simulink model "scdcstrctrlpidblock"  (Simulink 7.6)
settings: Solver=ode23s  StartTime=0  StopTime=60  RelTol=1e-3
libraries: simulink x1
settings Model: Creator=The MathWorks Inc.  BufferReuse=off
settings DataIOCC: InitialState=[311.267; 8.5695]  SaveOutput=off  SignalLogging=off  SaveTime=off  SignalLoggingName=logsOut
settings OptimizationCC: BooleanDataType=off  InlineParams=on  InlineInvariantSignals=on  BufferReuse=off  InitFltsAndDblsToZero=on
settings DebuggingCC: SaveWithParameterizedLinksMsg=none  CheckExecutionContextPreStartOutputMsg=on  CheckExecutionContextRuntimeOutputMsg=on  SignalResolutionControl=TryResolveAllWithWarning  SolverPrmCheckMsg=none  MultiTaskDSMMsg=warning  MultiTaskCondExecSysMsg=none  StrictBusMsg=None
settings HardwareCC: TargetUnknown=on
settings RTWCC: IncludeERTFirstTime=on
settings GRTTargetCC: TargetFcnLib=ansi_tfl_tmw.mat

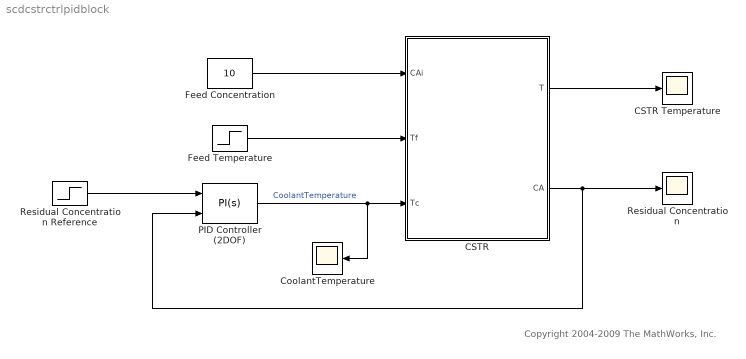
== system scdcstrctrlpidblock ==
  note: Copyright 2004-2009 The MathWorks, Inc.
  CSTR : Subsystem
  CSTR Temperature : Scope
      settings: YMin=300  YMax=750  SaveName=ScopeData2
  CoolantTemperature : Scope
      settings: YMin=300  YMax=750
  Feed Concentration : Constant  Value=10
  Feed Temperature : Step  Time=30  Before=300  After=305  SampleTime=0
  PID Controller (2DOF) : simulink/Continuous/PID Controller (2DOF)  DialogController=pidpack.PIDConfig.pidDDGCreate  DialogControllerArgs=DataTag0  SystemSampleTime=-1  Controller=PI  TimeDomain=Continuous-time  SampleTime=1  IntegratorMethod=Forward Euler  FilterMethod=Forward Euler  Form=Parallel  P=1  I=1  D=0  N=100  b=1  c=1  InitialConditionSource=internal  InitialConditionForIntegrator=300  InitialConditionForFilter=0  ExternalReset=none  ZeroCross=off  LimitOutput=off  UpperSaturationLimit=inf  LowerSaturationLimit=-inf  LinearizeAsGain=off  AntiWindupMode=none  Kb=1  TrackingMode=off  Kt=1  PParamMin=[ ]  PParamMax=[ ]  IParamMin=[ ]  IParamMax=[ ]  DParamMin=[ ]  DParamMax=[ ]  NParamMin=[ ]  NParamMax=[ ]  bParamMin=[ ]  bParamMax=[ ]  cParamMin=[ ]  cParamMax=[ ]  KbParamMin=[ ]  KbParamMax=[ ]  KtParamMin=[ ]  KtParamMax=[ ]  POutMin=[ ]  POutMax=[ ]  IOutMin=[ ]  IOutMax=[ ]  DOutMin=[ ]  DOutMax=[ ]  NOutMin=[ ]  NOutMax=[ ]  bOutMin=[ ]  bOutMax=[ ]  cOutMin=[ ]  cOutMax=[ ]  KbOutMin=[ ]  KbOutMax=[ ]  KtOutMin=[ ]  KtOutMax=[ ]  IntegratorOutMin=[ ]  IntegratorOutMax=[ ]  FilterOutMin=[ ]  FilterOutMax=[ ]  SumOutMin=[ ]  SumOutMax=[ ]  Sum1OutMin=[ ]  Sum1OutMax=[ ]  Sum2OutMin=[ ]  Sum2OutMax=[ ]  Sum3OutMin=[ ]  Sum3OutMax=[ ]  SumI1OutMin=[ ]  SumI1OutMax=[ ]  SumI2OutMin=[ ]  SumI2OutMax=[ ]  SumI3OutMin=[ ]  SumI3OutMax=[ ]  SumDOutMin=[ ]  SumDOutMax=[ ]  SaturationOutMin=[ ]  SaturationOutMax=[ ]  IntegratorContinuousStateAttributes=''  IntegratorStateMustResolveToSignalObject=off  IntegratorRTWStateStorageClass=Auto  FilterContinuousStateAttributes=''  FilterStateMustResolveToSignalObject=off  FilterRTWStateStorageClass=Auto
  Residual Concentration : Scope
      settings: YMin=0  YMax=9
  Residual Concentration Reference : Step  Time=2  Before=1.96  After=1.46  SampleTime=0
  wires:
  Feed Temperature/1 -> CSTR/2(Tf)
  CSTR/1(T) -> CSTR Temperature/1
  Feed Concentration/1 -> CSTR/1(CAi)
  PID Controller (2DOF)/1 -> CSTR/3(Tc), CoolantTemperature/1  "CoolantTemperature"
  Residual Concentration Reference/1 -> PID Controller (2DOF)/1
  CSTR/2(CA) -> Residual Concentration/1, PID Controller (2DOF)/2

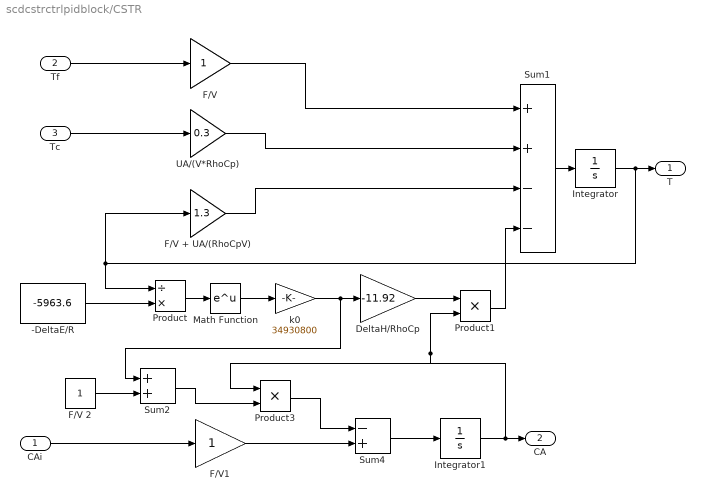
== system scdcstrctrlpidblock/CSTR ==
  CAi : Inport
  Tf : Inport  Port=2
  Tc : Inport  Port=3
  -DeltaE/R : Constant  Value=-5963.6
  DeltaH/RhoCp : Gain  Gain=-11.92  SaturateOnIntegerOverflow=on  OutDataTypeStr=Inherit: Same as input  ParamDataTypeStr=Inherit: Same as input
  F/V : Gain  SaturateOnIntegerOverflow=on  OutDataTypeStr=Inherit: Same as input  ParamDataTypeStr=Inherit: Same as input
  F/V + UA/(RhoCpV) : Gain  Gain=1.3  SaturateOnIntegerOverflow=on  OutDataTypeStr=Inherit: Same as input  ParamDataTypeStr=Inherit: Same as input
  F/V 2 : Constant
  F/V1 : Gain  SaturateOnIntegerOverflow=on  OutDataTypeStr=Inherit: Same as input  ParamDataTypeStr=Inherit: Same as input
  Integrator : Integrator  InitialCondition=373.7214  LimitOutput=on  LowerSaturationLimit=0
  Integrator1 : Integrator  InitialCondition=1.96  LimitOutput=on  LowerSaturationLimit=0
  Math Function : Math  SaturateOnIntegerOverflow=on
  Product : Product  Inputs=/*  SaturateOnIntegerOverflow=on  RndMeth=Zero  InputSameDT=on  OutDataTypeStr=Inherit: Same as first input
  Product1 : Product  SaturateOnIntegerOverflow=on  RndMeth=Zero  InputSameDT=on  OutDataTypeStr=Inherit: Same as first input
  Product3 : Product  SaturateOnIntegerOverflow=on  RndMeth=Zero  InputSameDT=on  OutDataTypeStr=Inherit: Same as first input
  Sum1 : Sum  Inputs=++--  SaturateOnIntegerOverflow=on  InputSameDT=on  OutDataTypeStr=Inherit: Same as first input
  Sum2 : Sum  SaturateOnIntegerOverflow=on  InputSameDT=on  OutDataTypeStr=Inherit: Same as first input
  Sum4 : Sum  Inputs=-+  SaturateOnIntegerOverflow=on  InputSameDT=on  OutDataTypeStr=Inherit: Same as first input
  UA/(V*RhoCp) : Gain  Gain=0.3  SaturateOnIntegerOverflow=on  OutDataTypeStr=Inherit: Same as input  ParamDataTypeStr=Inherit: Same as input
  k0 : Gain  Gain=34930800  SaturateOnIntegerOverflow=on  OutDataTypeStr=Inherit: Same as input  ParamDataTypeStr=Inherit: Same as input
  T : Outport
  CA : Outport  Port=2
  wires:
  F/V/1 -> Sum1/1
  Sum1/1 -> Integrator/1
  Integrator/1 -> Product/1, F/V + UA/(RhoCpV)/1, T/1
  UA/(V*RhoCp)/1 -> Sum1/2
  F/V + UA/(RhoCpV)/1 -> Sum1/3
  Product/1 -> Math Function/1
  Math Function/1 -> k0/1
  DeltaH/RhoCp/1 -> Product1/1
  Product1/1 -> Sum1/4
  k0/1 -> DeltaH/RhoCp/1, Sum2/1
  -DeltaE/R/1 -> Product/2
  Product3/1 -> Sum4/1
  Sum4/1 -> Integrator1/1
  Integrator1/1 -> Product3/1, Product1/2, CA/1
  F/V 2/1 -> Sum2/2
  F/V1/1 -> Sum4/2
  Tf/1 -> F/V/1
  CAi/1 -> F/V1/1
  Tc/1 -> UA/(V*RhoCp)/1
  Sum2/1 -> Product3/2
